simulink model "case3"  (Simulink 6.6)
settings: Solver=ode45  StartTime=0.0  StopTime=36  RelTol=1e-3
undefined symbols (not defined in the file or in its folder): sigbuilder_block
settings Model: Creator=MXKana  LastModifiedBy=mxkana

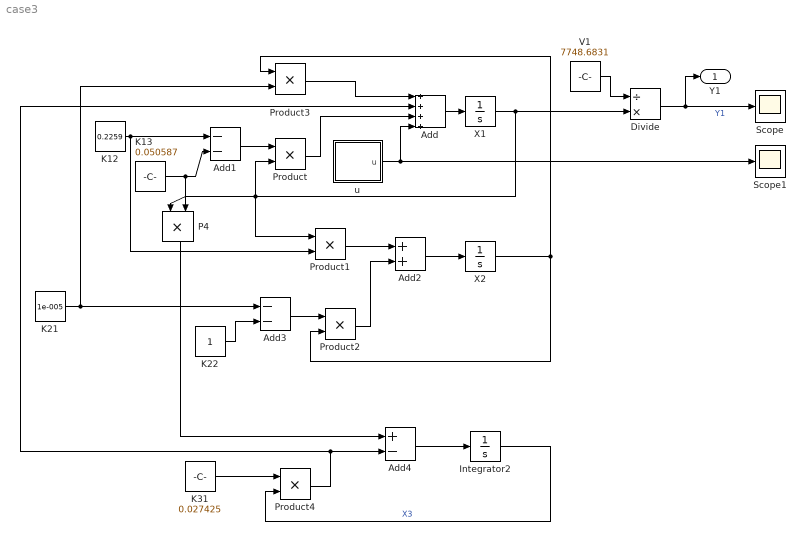
== system case3 ==
  Add : Sum  Inputs=++++  OutScaling=2^-10
  Add1 : Sum  Inputs=--  OutScaling=2^-10
  Add2 : Sum  OutScaling=2^-10
  Add3 : Sum  Inputs=--  OutScaling=2^-10
  Add4 : Sum  Inputs=+-  OutScaling=2^-10
  Divide : Product  Inputs=/*  OutScaling=2^-10
  Integrator2 : Integrator
  K12 : Constant  Value=0.2259
  K13 : Constant  Value=0.050587
  K21 : Constant  Value=1e-005
  K22 : Constant
  K31 : Constant  Value=0.027425
  P4 : Product  Orientation=down  RndMeth=Zero
  Product{,1..4} (5 alike) : Product  RndMeth=Zero
  Scope : Scope
  Scope1 : Scope
  V1 : Constant  Value=7748.6831
  X1 : Integrator
  X2 : Integrator
  u : Subsystem  Tag=STV Subsys  LoadFcn=sigbuilder_block('load',[406.5 183 550.5 363.75 ]);  StartFcn=sigbuilder_block('start');  StopFcn=sigbuilder_block('stop');  ClipboardFcn=sigbuilder_block('clipboard');  mask(Sigbuilder block){}
      mask help: Sigbuilder GUI
      mask init:
      | if ~strcmp(get_param(bdroot(gcbh),'SimulationStatus'),'stopped') tuvar = sigbuilder_block('maskInit'); end
      settings: CopyFcn=sigbuilder_block('copy');  DeleteFcn=sigbuilder_block('delete');  ModelCloseFcn=sigbuilder_block('modelClose');  PreSaveFcn=sigbuilder_block('preSave');  NameChangeFcn=sigbuilder_block('namechange');  OpenFcn=sigbuilder_block('open',[406.5 183 550.5 363.75 ]);  CloseFcn=sigbuilder_block('close');
      mask Display: plot(0,0,100,100,[10,10,40,40,10],[80,20,20,80,80],[40,10],[50,50], [40,27,10],[65,72,56],[40,25,25,10],[28,28,43,43]);
  Y1 : Outport
  wires:
  Add/1 -> X1/1
  K12/1 -> Add1/1, Product1/2
  K13/1 -> Add1/2, P4/1
  X1/1 -> Product1/1, Product/2, P4/2, Divide/2
  Add2/1 -> X2/1
  Product1/1 -> Add2/1
  K21/1 -> Add3/1, Product3/2
  K22/1 -> Add3/2
  Add3/1 -> Product2/1
  X2/1 -> Product2/2, Product3/1
  Product2/1 -> Add2/2
  Add1/1 -> Product/1
  Product/1 -> Add/3
  Add4/1 -> Integrator2/1
  K31/1 -> Product4/1
  P4/1 -> Add4/1
  Product4/1 -> Add4/2, Add/2
  Integrator2/1 -> Product4/2  "X3"
  Product3/1 -> Add/1
  Divide/1 -> Y1/1, Scope/1  "Y1"
  u/1(u) -> Add/4, Scope1/1
  V1/1 -> Divide/1

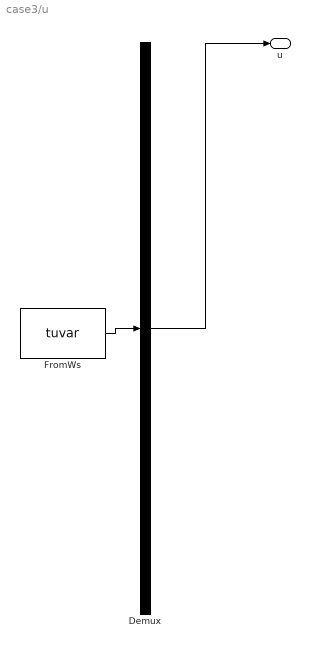
== system case3/u ==
  Demux : Demux  Tag=STV Demux  Outputs=1
  FromWs : FromWorkspace  Tag=STV FromWs  VariableName=tuvar  SampleTime=0  SigBuilderData=DataTag0  VnvData=DataTag1
      SigBuilderData=|
      | channels.label = 'u'
      | channels.allXData = {[0 1 1 36]}
      | channels.allYData = {[100000 100000 0 0]}
      | common.afterFinalStr = 'Extrapolate'
      | common.sampleTime = 0
      | dataSet.timeRange = [0 36]
      | dataSet.name = 'Group 1'
  u : Outport  Tag=STV Outport
  wires:
  Demux/1 -> u/1
  FromWs/1 -> Demux/1
